simulink model "XM7p_new"  (R2024a)
settings: Solver=ode4  StartTime=0.0  StopTime=60  RelTol=1e-3
model workspace (MAT data in the model file):
  a_value = 1
undefined symbols (not defined in the file or in its folder): a, b, c_pol, dt, traj_par, X, Y, Z
libraries: sm_lib x280, nesl_utility x109, simulink x14
(part 1 of 6)
settings Model: Creator=asus  LastModifiedBy=17599
settings DebuggingCC: UnconnectedInputMsg=warning  UnconnectedOutputMsg=warning  UnconnectedLineMsg=warning
settings ModelReferenceCC: EnableRefExpFcnMdlSchedulingChecks=on
settings RTWCC: GPUComputeCapability=3.5  DLArmComputeVersion=19.05
settings ExplorerConfigSet: InternalSimMechanicsExplorerSettings="<ExplorerConfiguration><canonicalview>default</canonicalview><AnimationSetting><BasePlaybackSpeed>1.0</BasePlaybackSpeed><PlaybackSpeedFactor>1.0</PlaybackSpeedFactor></AnimationSetting><TilePanel><TileInfo><Tiles Columns=\"1\" Count=\"1\" Rows=\"1\"><Column Weight=\"1\"/><Row Weight=\"1\"/><Tile Height=\"1\" Width=\"1\" X=\"0\" Y=\"0\"/></Tiles></TileInfo><SceneInfo><SceneViewer><BGColor><R>0.60000002384185791</R><G>0.60000002384185791</G><B>0.60000002384185791</B></BGColor><Camera><DoPerspective>off</DoPerspective><Position><X>0.201838941505270653</X><Y>-1.16911856832824412</Y><Z>0.702483401800660268</Z></Position><Center><X>0.1539467503897545</X><Y>0.000995467000701073627</Y><Z>0.7153569470392378</Z></Center><Up><X>0.00490593321745084673</X><Y>-0.0108003862646076643</Y><Z>0.999929639262584158</Z></Up><ViewLimDist>1</ViewLimDist><YLim>0.987066108097597317</YLim><XLim>1.59392897455760174</XLim></Camera></SceneViewer></SceneInfo></TilePanel><MechEditorPanel><Cameras/><GfxPanelCameraMap/><VideoCreator><PlaybackSpeedRatio>1.0</PlaybackSpeedRatio><FrameRate>30</FrameRate><VideoFormat>MPEG-4</VideoFormat><FrameSize>auto</FrameSize></VideoCreator></MechEditorPanel></ExplorerConfiguration>"

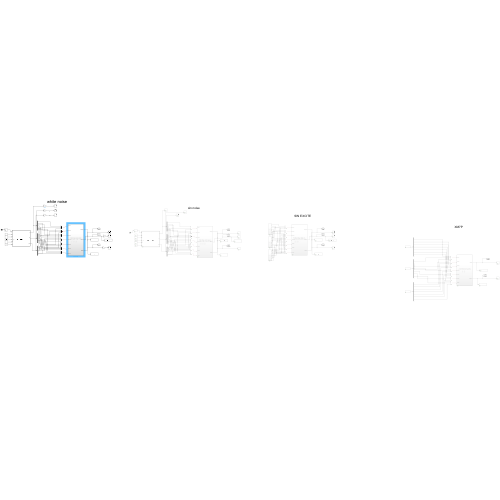
[thumbnail: Simulink's stored preview of the top-level diagram]
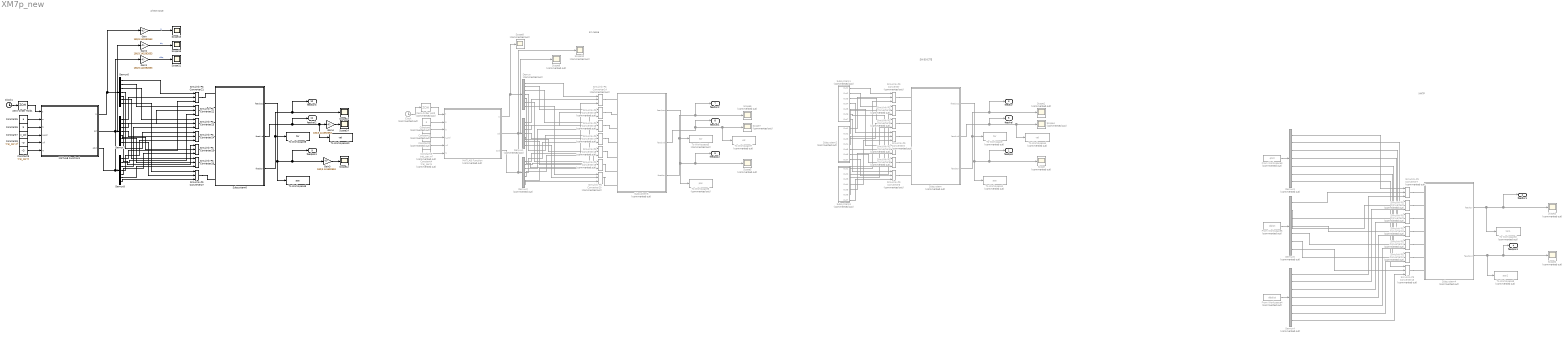
== system XM7p_new ==
  note: SIN EXCITE
  note: XM7P
  note: sin noise
  note: white noise
  Clock : Clock  Commented=on
  Clock1 : Clock
  Constant : Constant  Commented=on  Value=a  VectorParams1D=off
  Constant1 : Constant  Commented=on  Value=b  VectorParams1D=off
  Constant2 : Constant  Commented=on  Value=c_pol  VectorParams1D=off
  Constant3 : Constant  Commented=on  Value=traj_par.wf  VectorParams1D=off
  Constant4 : Constant  Commented=on  Value=traj_par.N  VectorParams1D=off
  Constant5 : Constant  Value=a  VectorParams1D=off
  Constant6 : Constant  Value=b  VectorParams1D=off
  Constant7 : Constant  Value=c_pol  VectorParams1D=off
  Constant8 : Constant  Value=traj_par.wf  VectorParams1D=off
  Constant9 : Constant  Value=traj_par.N  VectorParams1D=off
  Demux{,1..5} (6 alike) : Demux  Commented=on  Outputs=7
  Demux6 : Demux  Outputs=7
  Demux7 : Demux  Outputs=7
  Demux8 : Demux  Outputs=7
  From Workspace3 : FromWorkspace  Commented=on  VariableName=qlist  SampleTime=dt
  From Workspace4 : FromWorkspace  Commented=on  VariableName=ddqlist  SampleTime=dt
  From Workspace5 : FromWorkspace  Commented=on  VariableName=dqlist  SampleTime=dt
  Gain{,1..4} (5 alike) : Gain  Gain=180/3.141592653
  MATLAB Function : MATLAB Function  Commented=on  TreatAsAtomicUnit=on
  MATLAB Function1 : MATLAB Function  TreatAsAtomicUnit=on
  Scope{,1..10} (11 alike) : Scope  Commented=on
  Scope{11..16} (6 alike) : Scope
  Simulink-PS Converter{,1..20} (21 alike) : nesl_utility/Simulink-PS Converter  Commented=on  PhysicalDomain=network_engine_domain  SubClassName=ps_input  LeftPortType=input  RightPortType=output  PseudoPeriodic=off  Frequencies=[]  NoiseDistribution=none  NoiseParameters=[]  Unit=rad  AffineConversion=off  FilteringAndDerivatives=provide  SimscapeFilterOrder=2  InputFilterTimeConstant=0.001  UdotUserProvided=2
  Simulink-PS Converter{21..27} (7 alike) : nesl_utility/Simulink-PS Converter  PhysicalDomain=network_engine_domain  SubClassName=ps_input  LeftPortType=input  RightPortType=output  PseudoPeriodic=off  Frequencies=[]  NoiseDistribution=none  NoiseParameters=[]  Unit=rad  AffineConversion=off  FilteringAndDerivatives=provide  SimscapeFilterOrder=2  InputFilterTimeConstant=0.001  UdotUserProvided=2
  Subsystem : Subsystem  Commented=on
  Subsystem1 : Subsystem  Commented=on
  Subsystem2 : Subsystem  Commented=on
  Subsystem3 : Subsystem  Commented=on
  Subsystem4 : Subsystem  Commented=on
  Subsystem5 : Subsystem  Commented=on
  Subsystem6 : Subsystem
  To Workspace : ToWorkspace  Commented=on  VariableName=tor  SampleTime=-1
      settings: Save2DSignal=2-D array (concatenate along first dimension)
  To Workspace1 : ToWorkspace  Commented=on  VariableName=pos  SampleTime=-1
      settings: Save2DSignal=2-D array (concatenate along first dimension)
  To Workspace10 : ToWorkspace  VariableName=vel  SampleTime=-1
      settings: Save2DSignal=2-D array (concatenate along first dimension)
  To Workspace2 : ToWorkspace  Commented=on  VariableName=tor1  SampleTime=-1
      settings: Save2DSignal=2-D array (concatenate along first dimension)
  To Workspace3 : ToWorkspace  Commented=on  VariableName=pos1  SampleTime=-1
      settings: Save2DSignal=2-D array (concatenate along first dimension)
  To Workspace4 : ToWorkspace  Commented=on  VariableName=vel  SampleTime=-1
      settings: Save2DSignal=2-D array (concatenate along first dimension)
  To Workspace5 : ToWorkspace  Commented=on  VariableName=tor  SampleTime=-1
      settings: Save2DSignal=2-D array (concatenate along first dimension)
  To Workspace6 : ToWorkspace  Commented=on  VariableName=pos  SampleTime=-1
      settings: Save2DSignal=2-D array (concatenate along first dimension)
  To Workspace7 : ToWorkspace  Commented=on  VariableName=vel  SampleTime=-1
      settings: Save2DSignal=2-D array (concatenate along first dimension)
  To Workspace8 : ToWorkspace  VariableName=tor  SampleTime=-1
      settings: Save2DSignal=2-D array (concatenate along first dimension)
  To Workspace9 : ToWorkspace  VariableName=pos  SampleTime=-1
      settings: Save2DSignal=2-D array (concatenate along first dimension)
  Zero-Order Hold : ZeroOrderHold  Commented=on  SampleTime=0.001
  Zero-Order Hold1 : ZeroOrderHold  SampleTime=0.001
  feedpos : Outport  Unit=rad
  feedtor1 : Outport  Port=2  Unit=N*m
  feedtor : Outport  Port=3  Unit=N*m
  feedpos1 : Outport  Port=4  Unit=rad
  feedvel : Outport  Port=5  Unit=rad/s
  feedpos2 : Outport  Port=6  Unit=rad
  feedtor2 : Outport  Port=7  Unit=N*m
  feedvel1 : Outport  Port=8  Unit=rad/s
  feedpos3 : Outport  Port=9  Unit=rad
  feedtor3 : Outport  Port=10  Unit=N*m
  feedvel2 : Outport  Port=11  Unit=rad/s
  wires:
  Subsystem/3(feedtor) -> feedtor/1, Scope1/1, To Workspace/1
  Subsystem/1(feedpos) -> To Workspace1/1, feedpos/1, Scope/1
  Subsystem1/1(Out1) -> Simulink-PS Converter/1
  Subsystem1/2(Out2) -> Simulink-PS Converter1/1
  Subsystem1/3(Out3) -> Simulink-PS Converter2/1
  Subsystem1/4(Out4) -> Simulink-PS Converter3/1
  Subsystem1/5(Out5) -> Simulink-PS Converter4/1
  Subsystem1/6(Out6) -> Simulink-PS Converter5/1
  Subsystem1/7(Out7) -> Simulink-PS Converter6/1
  Subsystem2/1(Out1) -> Simulink-PS Converter/2
  Subsystem2/2(Out2) -> Simulink-PS Converter1/2
  Subsystem2/3(Out3) -> Simulink-PS Converter2/2
  Subsystem2/4(Out4) -> Simulink-PS Converter3/2
  Subsystem2/5(Out5) -> Simulink-PS Converter4/2
  Subsystem2/6(Out6) -> Simulink-PS Converter5/2
  Subsystem2/7(Out7) -> Simulink-PS Converter6/2
  Subsystem3/1(Out1) -> Simulink-PS Converter/3
  Subsystem3/2(Out2) -> Simulink-PS Converter1/3
  Subsystem3/3(Out3) -> Simulink-PS Converter2/3
  Subsystem3/4(Out4) -> Simulink-PS Converter3/3
  Subsystem3/5(Out5) -> Simulink-PS Converter4/3
  Subsystem3/6(Out6) -> Simulink-PS Converter5/3
  Subsystem3/7(Out7) -> Simulink-PS Converter6/3
  Demux3/5 -> Simulink-PS Converter11/1
  Demux4/6 -> Simulink-PS Converter12/3
  Demux5/2 -> Simulink-PS Converter8/2
  Demux4/5 -> Simulink-PS Converter11/3
  Demux5/7 -> Simulink-PS Converter13/2
  Demux5/3 -> Simulink-PS Converter9/2
  Demux4/7 -> Simulink-PS Converter13/3
  Demux3/2 -> Simulink-PS Converter8/1
  Demux3/4 -> Simulink-PS Converter10/1
  From Workspace5/1 -> Demux5/1
  Demux4/3 -> Simulink-PS Converter9/3
  Demux5/5 -> Simulink-PS Converter11/2
  Demux3/3 -> Simulink-PS Converter9/1
  Subsystem4/2(feedpos) -> Scope2/1, feedpos1/1, To Workspace3/1
  Demux4/2 -> Simulink-PS Converter8/3
  Demux4/1 -> Simulink-PS Converter7/3
  Demux4/4 -> Simulink-PS Converter10/3
  Demux3/6 -> Simulink-PS Converter12/1
  From Workspace3/1 -> Demux3/1
  Demux5/6 -> Simulink-PS Converter12/2
  From Workspace4/1 -> Demux4/1
  Demux5/4 -> Simulink-PS Converter10/2
  Demux3/1 -> Simulink-PS Converter7/1
  Demux5/1 -> Simulink-PS Converter7/2
  Subsystem4/1(feedtor) -> To Workspace2/1, feedtor1/1, Scope3/1
  Demux3/7 -> Simulink-PS Converter13/1
  Subsystem/2(feedvel) -> feedvel/1, To Workspace4/1, Scope4/1
  Subsystem5/2(feedvel) -> feedvel1/1, To Workspace7/1, Scope7/1
  Subsystem5/1(feedpos) -> To Workspace6/1, feedpos2/1, Scope5/1
  Subsystem5/3(feedtor) -> feedtor2/1, Scope6/1, To Workspace5/1
  Clock/1 -> Zero-Order Hold/1
  Constant/1 -> MATLAB Function/2(a)
  Constant1/1 -> MATLAB Function/3(b)
  Constant2/1 -> MATLAB Function/4(c_pol)
  Constant3/1 -> MATLAB Function/5(wf)
  Constant4/1 -> MATLAB Function/6(N)
  Demux/1 -> Simulink-PS Converter14/1
  Demux/2 -> Simulink-PS Converter15/1
  Demux/3 -> Simulink-PS Converter16/1
  Demux/4 -> Simulink-PS Converter17/1
  Demux/5 -> Simulink-PS Converter18/1
  Demux/6 -> Simulink-PS Converter19/1
  Demux/7 -> Simulink-PS Converter20/1
  Demux1/1 -> Simulink-PS Converter14/2
  Demux1/2 -> Simulink-PS Converter15/2
  Demux1/3 -> Simulink-PS Converter16/2
  Demux1/4 -> Simulink-PS Converter17/2
  Demux1/5 -> Simulink-PS Converter18/2
  Demux1/6 -> Simulink-PS Converter19/2
  Demux1/7 -> Simulink-PS Converter20/2
  Demux2/1 -> Simulink-PS Converter14/3
  Demux2/2 -> Simulink-PS Converter15/3
  Demux2/3 -> Simulink-PS Converter16/3
  Demux2/4 -> Simulink-PS Converter17/3
  Demux2/5 -> Simulink-PS Converter18/3
  Demux2/6 -> Simulink-PS Converter19/3
  Demux2/7 -> Simulink-PS Converter20/3
  MATLAB Function/1(q) -> Scope8/1, Demux/1
  MATLAB Function/2(qd) -> Scope9/1, Demux1/1
  MATLAB Function/3(q2d) -> Scope10/1, Demux2/1
  Zero-Order Hold/1 -> MATLAB Function/1(t)
  Demux7/3 -> Simulink-PS Converter23/2
  Demux7/4 -> Simulink-PS Converter24/2
  Constant8/1 -> MATLAB Function1/5(wf)
  Subsystem6/3(feedtor) -> feedtor3/1, Scope13/1, To Workspace8/1
  Clock1/1 -> Zero-Order Hold1/1
  Constant9/1 -> MATLAB Function1/6(N)
  Demux6/7 -> Simulink-PS Converter27/1
  Demux6/6 -> Simulink-PS Converter26/1
  Demux6/4 -> Simulink-PS Converter24/1
  Demux7/1 -> Simulink-PS Converter21/2
  Demux6/5 -> Simulink-PS Converter25/1
  Demux7/5 -> Simulink-PS Converter25/2
  Subsystem6/1(feedpos) -> To Workspace9/1, feedpos3/1, Gain3/1
  Zero-Order Hold1/1 -> MATLAB Function1/1(t)
  MATLAB Function1/2(qd) -> Gain2/1, Demux7/1
  Demux8/1 -> Simulink-PS Converter21/3
  Demux6/2 -> Simulink-PS Converter22/1
  MATLAB Function1/3(q2d) -> Gain1/1, Demux8/1
  Subsystem6/2(feedvel) -> feedvel2/1, To Workspace10/1, Gain4/1
  Demux8/7 -> Simulink-PS Converter27/3
  Demux6/1 -> Simulink-PS Converter21/1
  Constant7/1 -> MATLAB Function1/4(c_pol)
  MATLAB Function1/1(q) -> Gain/1, Demux6/1
  Demux8/2 -> Simulink-PS Converter22/3
  Demux8/3 -> Simulink-PS Converter23/3
  Demux8/5 -> Simulink-PS Converter25/3
  Demux8/6 -> Simulink-PS Converter26/3
  Demux7/2 -> Simulink-PS Converter22/2
  Constant5/1 -> MATLAB Function1/2(a)
  Demux7/7 -> Simulink-PS Converter27/2
  Constant6/1 -> MATLAB Function1/3(b)
  Demux6/3 -> Simulink-PS Converter23/1
  Demux8/4 -> Simulink-PS Converter24/3
  Demux7/6 -> Simulink-PS Converter26/2
  Gain/1 -> Scope15/1  "q"
  Gain1/1 -> Scope11/1  "ddq"
  Gain2/1 -> Scope16/1  "dq"
  Gain3/1 -> Scope12/1
  Gain4/1 -> Scope14/1
  connections:
  Simulink-PS Converter/RConn1 -- Subsystem/LConn1
  Simulink-PS Converter6/RConn1 -- Subsystem/LConn7
  Simulink-PS Converter4/RConn1 -- Subsystem/LConn5
  Simulink-PS Converter2/RConn1 -- Subsystem/LConn3
  Simulink-PS Converter1/RConn1 -- Subsystem/LConn2
  Simulink-PS Converter5/RConn1 -- Subsystem/LConn6
  Simulink-PS Converter3/RConn1 -- Subsystem/LConn4
  Simulink-PS Converter10/RConn1 -- Subsystem4/LConn4
  Simulink-PS Converter13/RConn1 -- Subsystem4/LConn7
  Simulink-PS Converter9/RConn1 -- Subsystem4/LConn3
  Simulink-PS Converter8/RConn1 -- Subsystem4/LConn2
  Simulink-PS Converter12/RConn1 -- Subsystem4/LConn6
  Simulink-PS Converter7/RConn1 -- Subsystem4/LConn1
  Simulink-PS Converter11/RConn1 -- Subsystem4/LConn5
  Simulink-PS Converter14/RConn1 -- Subsystem5/LConn1
  Simulink-PS Converter20/RConn1 -- Subsystem5/LConn7
  Simulink-PS Converter17/RConn1 -- Subsystem5/LConn4
  Simulink-PS Converter18/RConn1 -- Subsystem5/LConn5
  Simulink-PS Converter19/RConn1 -- Subsystem5/LConn6
  Simulink-PS Converter15/RConn1 -- Subsystem5/LConn2
  Simulink-PS Converter16/RConn1 -- Subsystem5/LConn3
  Simulink-PS Converter26/RConn1 -- Subsystem6/LConn6
  Simulink-PS Converter22/RConn1 -- Subsystem6/LConn2
  Simulink-PS Converter27/RConn1 -- Subsystem6/LConn7
  Simulink-PS Converter24/RConn1 -- Subsystem6/LConn4
  Simulink-PS Converter23/RConn1 -- Subsystem6/LConn3
  Simulink-PS Converter25/RConn1 -- Subsystem6/LConn5
  Simulink-PS Converter21/RConn1 -- Subsystem6/LConn1

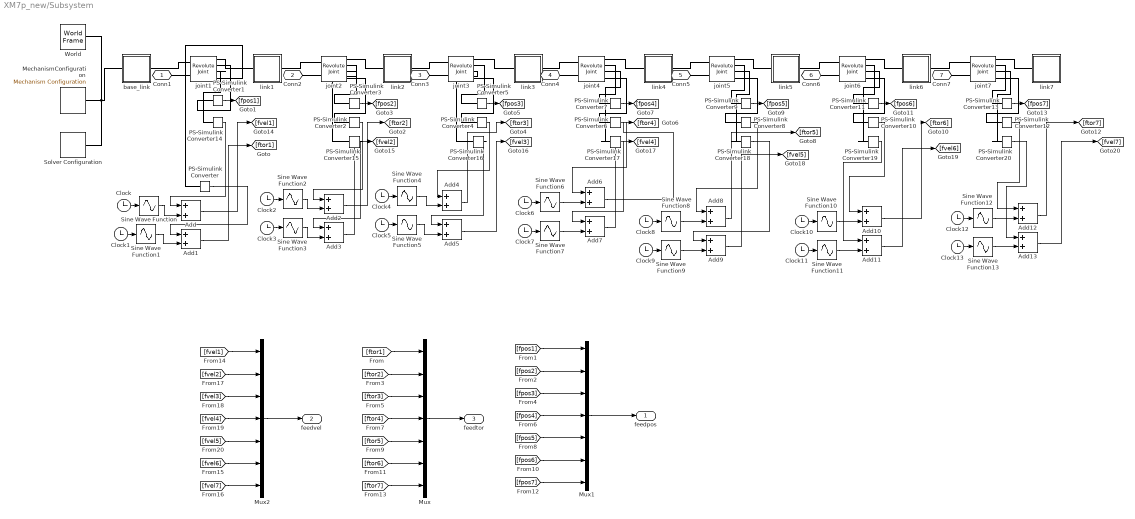
== system XM7p_new/Subsystem ==
  Add{,1..13} (14 alike) : Sum
  Clock{,1..13} (14 alike) : Clock
  MechanismConfiguration : sm_lib/Utilities/Mechanism Configuration  UniformGravity=Constant  GravityVector=[0 0 -9.80665]  GravityVectorUnits=m/s^2  LinearizationDelta=0.001  JointModeTransitionNonlinearIterations=2
  Mux : Mux  Inputs=7
  Mux1 : Mux  Inputs=7
  Mux2 : Mux  Inputs=7
  PS-Simulink Converter{,2,4,6,8,10,12} (7 alike) : nesl_utility/PS-Simulink Converter  PhysicalDomain=network_engine_domain  SubClassName=ps_output  LeftPortType=input  RightPortType=output  PseudoPeriodic=off  Frequencies=[]  VectorFormat=1-D array  Unit=N*m  AffineConversion=off
  PS-Simulink Converter{1,3,5,7,9,11,13} (7 alike) : nesl_utility/PS-Simulink Converter  PhysicalDomain=network_engine_domain  SubClassName=ps_output  LeftPortType=input  RightPortType=output  PseudoPeriodic=off  Frequencies=[]  VectorFormat=1-D array  Unit=rad  AffineConversion=off
  PS-Simulink Converter{14..20} (7 alike) : nesl_utility/PS-Simulink Converter  PhysicalDomain=network_engine_domain  SubClassName=ps_output  LeftPortType=input  RightPortType=output  PseudoPeriodic=off  Frequencies=[]  VectorFormat=1-D array  Unit=rad/s  AffineConversion=off
  Sine Wave Function{,1,3..5} (5 alike) : Sin  TimeSource=Use external signal  Amplitude=0.05  Frequency=10  SampleTime=0
  Sine Wave Function{6..11} (6 alike) : Sin  TimeSource=Use external signal  Amplitude=0.03  Frequency=10  SampleTime=0
  Sine Wave Function12 : Sin  TimeSource=Use external signal  Amplitude=0.02  Frequency=10  SampleTime=0
  Sine Wave Function13 : Sin  TimeSource=Use external signal  Amplitude=0.02  Frequency=10  SampleTime=0
  Sine Wave Function2 : Sin  TimeSource=Use external signal  Amplitude=0.05  SampleTime=0
  Solver Configuration : nesl_utility/Solver Configuration  PhysicalDomain=network_engine_domain  SubClassName=solver  LeftPortType=input  RightPortType=generic  Tones=[]  Harmonics=[]  SimulateNoise=off  Profile=off  UseLocalSampling=off  EnableSwitchedLinearOptims=on  FrequencyDomain=off  UseCCode=off  RelTol=0.001  AbsTol=1e-06  MinStep=1e-09  ToWorkspace=off  RevertToSquareIcSolve=off  NumHomotopyIterations=100  PhasorMode=off  PhasorModeNumHarmonics=1  ConsistencySolver=NEWTON_FTOL  IndexReductionMethod=DerivativeReplacement  DoDC=off  ResidualTolerance=1e-09  ConsistencyTolSource=GLOBAL  ConsistencyAbsTol=0.001  ConsistencyRelTol=0.001  ConsistencyTolFactor=0.001  UseLocalSolver=off  LocalSolverChoice=NE_BACKWARD_EULER_ADVANCER  ResolveIndetEquations=on  FunctionEvalNumThread=1  LocalSolverSampleTime=0.001  DoFixedCost=off  MaxNonlinIter=3  MaxModeIter=2  ComputeImpulses=off  ImpulseIterations=2  LinearAlgebra=auto  LinearAlgebraNumThread=0  EquationFormulation=NE_TIME_EF  DelaysMemoryBudget=1024  AutomaticFiltering=on  FilteringTimeConstant=0.001  PartitionStorageMethod=AS_NEEDED  PartitionMemoryBudget=1024  PartitionMethod=ROBUST  MultibodyUseLocalSolver=off  MultibodyLocalSolverChoice=ODE1  MultibodyLocalSolverSampleTime=0.001
  World : sm_lib/Frames and Transforms/World Frame
  base_link : Subsystem
  joint1 : sm_lib/Joints/Revolute Joint  JointMode=Normal  CompositeWrenchDir=FollowerOnBase  CompositeWrenchFrame=BaseFrame  SenseConstraintForce=off  SenseConstraintTorque=off  SenseTotalForce=off  SenseTotalTorque=off  PositionTargetSpecify=off  PositionTargetPriority=High  PositionTargetValue=0  PositionTargetValueUnits=deg  VelocityTargetSpecify=off  VelocityTargetPriority=High  VelocityTargetValue=0  VelocityTargetValueUnits=deg/s  EquilibriumPosition=0  EquilibriumPositionUnits=deg  SpringStiffness=0  SpringStiffnessUnits=N*m/deg  DampingCoefficient=0  DampingCoefficientUnits=kg*m^2/(rad*s)  LowerLimitSpecify=on  LowerLimitBound=-3.1067  LowerLimitBoundUnits=rad  LowerLimitStiffness=1e4  LowerLimitStiffnessUnits=N*m/deg  LowerLimitDamping=10  LowerLimitDampingUnits=N*m/(deg/s)  LowerLimitTransitionRegionWidth=0.1  LowerLimitTransitionRegionWidthUnits=deg  UpperLimitSpecify=on  UpperLimitBound=3.1067  UpperLimitBoundUnits=rad  UpperLimitStiffness=1e4  UpperLimitStiffnessUnits=N*m/deg  UpperLimitDamping=10  UpperLimitDampingUnits=N*m/(deg/s)  UpperLimitTransitionRegionWidth=0.1  UpperLimitTransitionRegionWidthUnits=deg  TorqueActuationMode=ComputedTorque  MotionActuationMode=InputMotion  SensePosition=on  SenseVelocity=on  SenseAcceleration=off  SenseTorqueForce=on  SenseLowerLimitTorqueForce=off  SenseUpperLimitTorqueForce=off
  joint2 : sm_lib/Joints/Revolute Joint  JointMode=Normal  CompositeWrenchDir=FollowerOnBase  CompositeWrenchFrame=BaseFrame  SenseConstraintForce=off  SenseConstraintTorque=off  SenseTotalForce=off  SenseTotalTorque=off  PositionTargetSpecify=off  PositionTargetPriority=High  PositionTargetValue=0  PositionTargetValueUnits=deg  VelocityTargetSpecify=off  VelocityTargetPriority=High  VelocityTargetValue=0  VelocityTargetValueUnits=deg/s  EquilibriumPosition=0  EquilibriumPositionUnits=deg  SpringStiffness=0  SpringStiffnessUnits=N*m/deg  DampingCoefficient=0  DampingCoefficientUnits=kg*m^2/(rad*s)  LowerLimitSpecify=on  LowerLimitBound=-2.09  LowerLimitBoundUnits=rad  LowerLimitStiffness=1e4  LowerLimitStiffnessUnits=N*m/deg  LowerLimitDamping=10  LowerLimitDampingUnits=N*m/(deg/s)  LowerLimitTransitionRegionWidth=0.1  LowerLimitTransitionRegionWidthUnits=deg  UpperLimitSpecify=on  UpperLimitBound=2.09  UpperLimitBoundUnits=rad  UpperLimitStiffness=1e4  UpperLimitStiffnessUnits=N*m/deg  UpperLimitDamping=10  UpperLimitDampingUnits=N*m/(deg/s)  UpperLimitTransitionRegionWidth=0.1  UpperLimitTransitionRegionWidthUnits=deg  TorqueActuationMode=ComputedTorque  MotionActuationMode=InputMotion  SensePosition=on  SenseVelocity=on  SenseAcceleration=off  SenseTorqueForce=on  SenseLowerLimitTorqueForce=off  SenseUpperLimitTorqueForce=off
  joint3 : sm_lib/Joints/Revolute Joint  JointMode=Normal  CompositeWrenchDir=FollowerOnBase  CompositeWrenchFrame=BaseFrame  SenseConstraintForce=off  SenseConstraintTorque=off  SenseTotalForce=off  SenseTotalTorque=off  PositionTargetSpecify=off  PositionTargetPriority=High  PositionTargetValue=0  PositionTargetValueUnits=deg  VelocityTargetSpecify=off  VelocityTargetPriority=High  VelocityTargetValue=0  VelocityTargetValueUnits=deg/s  EquilibriumPosition=0  EquilibriumPositionUnits=deg  SpringStiffness=0  SpringStiffnessUnits=N*m/deg  DampingCoefficient=0  DampingCoefficientUnits=kg*m^2/(rad*s)  LowerLimitSpecify=on  LowerLimitBound=-3.1067  LowerLimitBoundUnits=rad  LowerLimitStiffness=1e4  LowerLimitStiffnessUnits=N*m/deg  LowerLimitDamping=10  LowerLimitDampingUnits=N*m/(deg/s)  LowerLimitTransitionRegionWidth=0.1  LowerLimitTransitionRegionWidthUnits=deg  UpperLimitSpecify=on  UpperLimitBound=3.1067  UpperLimitBoundUnits=rad  UpperLimitStiffness=1e4  UpperLimitStiffnessUnits=N*m/deg  UpperLimitDamping=10  UpperLimitDampingUnits=N*m/(deg/s)  UpperLimitTransitionRegionWidth=0.1  UpperLimitTransitionRegionWidthUnits=deg  TorqueActuationMode=ComputedTorque  MotionActuationMode=InputMotion  SensePosition=on  SenseVelocity=on  SenseAcceleration=off  SenseTorqueForce=on  SenseLowerLimitTorqueForce=off  SenseUpperLimitTorqueForce=off
  joint4 : sm_lib/Joints/Revolute Joint  JointMode=Normal  CompositeWrenchDir=FollowerOnBase  CompositeWrenchFrame=BaseFrame  SenseConstraintForce=off  SenseConstraintTorque=off  SenseTotalForce=off  SenseTotalTorque=off  PositionTargetSpecify=off  PositionTargetPriority=High  PositionTargetValue=0  PositionTargetValueUnits=deg  VelocityTargetSpecify=off  VelocityTargetPriority=High  VelocityTargetValue=0  VelocityTargetValueUnits=deg/s  EquilibriumPosition=0  EquilibriumPositionUnits=deg  SpringStiffness=0  SpringStiffnessUnits=N*m/deg  DampingCoefficient=0  DampingCoefficientUnits=kg*m^2/(rad*s)  LowerLimitSpecify=on  LowerLimitBound=-2.5307  LowerLimitBoundUnits=rad  LowerLimitStiffness=1e4  LowerLimitStiffnessUnits=N*m/deg  LowerLimitDamping=10  LowerLimitDampingUnits=N*m/(deg/s)  LowerLimitTransitionRegionWidth=0.1  LowerLimitTransitionRegionWidthUnits=deg  UpperLimitSpecify=on  UpperLimitBound=1.0472  UpperLimitBoundUnits=rad  UpperLimitStiffness=1e4  UpperLimitStiffnessUnits=N*m/deg  UpperLimitDamping=10  UpperLimitDampingUnits=N*m/(deg/s)  UpperLimitTransitionRegionWidth=0.1  UpperLimitTransitionRegionWidthUnits=deg  TorqueActuationMode=ComputedTorque  MotionActuationMode=InputMotion  SensePosition=on  SenseVelocity=on  SenseAcceleration=off  SenseTorqueForce=on  SenseLowerLimitTorqueForce=off  SenseUpperLimitTorqueForce=off
  joint5 : sm_lib/Joints/Revolute Joint  JointMode=Normal  CompositeWrenchDir=FollowerOnBase  CompositeWrenchFrame=BaseFrame  SenseConstraintForce=off  SenseConstraintTorque=off  SenseTotalForce=off  SenseTotalTorque=off  PositionTargetSpecify=off  PositionTargetPriority=High  PositionTargetValue=0  PositionTargetValueUnits=deg  VelocityTargetSpecify=off  VelocityTargetPriority=High  VelocityTargetValue=0  VelocityTargetValueUnits=deg/s  EquilibriumPosition=0  EquilibriumPositionUnits=deg  SpringStiffness=0  SpringStiffnessUnits=N*m/deg  DampingCoefficient=0  DampingCoefficientUnits=kg*m^2/(rad*s)  LowerLimitSpecify=on  LowerLimitBound=-3.1067  LowerLimitBoundUnits=rad  LowerLimitStiffness=1e4  LowerLimitStiffnessUnits=N*m/deg  LowerLimitDamping=10  LowerLimitDampingUnits=N*m/(deg/s)  LowerLimitTransitionRegionWidth=0.1  LowerLimitTransitionRegionWidthUnits=deg  UpperLimitSpecify=on  UpperLimitBound=3.1067  UpperLimitBoundUnits=rad  UpperLimitStiffness=1e4  UpperLimitStiffnessUnits=N*m/deg  UpperLimitDamping=10  UpperLimitDampingUnits=N*m/(deg/s)  UpperLimitTransitionRegionWidth=0.1  UpperLimitTransitionRegionWidthUnits=deg  TorqueActuationMode=ComputedTorque  MotionActuationMode=InputMotion  SensePosition=on  SenseVelocity=on  SenseAcceleration=off  SenseTorqueForce=on  SenseLowerLimitTorqueForce=off  SenseUpperLimitTorqueForce=off
  joint6 : sm_lib/Joints/Revolute Joint  JointMode=Normal  CompositeWrenchDir=FollowerOnBase  CompositeWrenchFrame=BaseFrame  SenseConstraintForce=off  SenseConstraintTorque=off  SenseTotalForce=off  SenseTotalTorque=off  PositionTargetSpecify=off  PositionTargetPriority=High  PositionTargetValue=0  PositionTargetValueUnits=deg  VelocityTargetSpecify=off  VelocityTargetPriority=High  VelocityTargetValue=0  VelocityTargetValueUnits=deg/s  EquilibriumPosition=0  EquilibriumPositionUnits=deg  SpringStiffness=0  SpringStiffnessUnits=N*m/deg  DampingCoefficient=0  DampingCoefficientUnits=kg*m^2/(rad*s)  LowerLimitSpecify=on  LowerLimitBound=-1.0472  LowerLimitBoundUnits=rad  LowerLimitStiffness=1e4  LowerLimitStiffnessUnits=N*m/deg  LowerLimitDamping=10  LowerLimitDampingUnits=N*m/(deg/s)  LowerLimitTransitionRegionWidth=0.1  LowerLimitTransitionRegionWidthUnits=deg  UpperLimitSpecify=on  UpperLimitBound=1.0472  UpperLimitBoundUnits=rad  UpperLimitStiffness=1e4  UpperLimitStiffnessUnits=N*m/deg  UpperLimitDamping=10  UpperLimitDampingUnits=N*m/(deg/s)  UpperLimitTransitionRegionWidth=0.1  UpperLimitTransitionRegionWidthUnits=deg  TorqueActuationMode=ComputedTorque  MotionActuationMode=InputMotion  SensePosition=on  SenseVelocity=on  SenseAcceleration=off  SenseTorqueForce=on  SenseLowerLimitTorqueForce=off  SenseUpperLimitTorqueForce=off
  joint7 : sm_lib/Joints/Revolute Joint  JointMode=Normal  CompositeWrenchDir=FollowerOnBase  CompositeWrenchFrame=BaseFrame  SenseConstraintForce=off  SenseConstraintTorque=off  SenseTotalForce=off  SenseTotalTorque=off  PositionTargetSpecify=off  PositionTargetPriority=High  PositionTargetValue=0  PositionTargetValueUnits=deg  VelocityTargetSpecify=off  VelocityTargetPriority=High  VelocityTargetValue=0  VelocityTargetValueUnits=deg/s  EquilibriumPosition=0  EquilibriumPositionUnits=deg  SpringStiffness=0  SpringStiffnessUnits=N*m/deg  DampingCoefficient=0  DampingCoefficientUnits=kg*m^2/(rad*s)  LowerLimitSpecify=on  LowerLimitBound=-1.5708  LowerLimitBoundUnits=rad  LowerLimitStiffness=1e4  LowerLimitStiffnessUnits=N*m/deg  LowerLimitDamping=10  LowerLimitDampingUnits=N*m/(deg/s)  LowerLimitTransitionRegionWidth=0.1  LowerLimitTransitionRegionWidthUnits=deg  UpperLimitSpecify=on  UpperLimitBound=1.5708  UpperLimitBoundUnits=rad  UpperLimitStiffness=1e4  UpperLimitStiffnessUnits=N*m/deg  UpperLimitDamping=10  UpperLimitDampingUnits=N*m/(deg/s)  UpperLimitTransitionRegionWidth=0.1  UpperLimitTransitionRegionWidthUnits=deg  TorqueActuationMode=ComputedTorque  MotionActuationMode=InputMotion  SensePosition=on  SenseVelocity=on  SenseAcceleration=off  SenseTorqueForce=on  SenseLowerLimitTorqueForce=off  SenseUpperLimitTorqueForce=off
  link1 : Subsystem
  link2 : Subsystem
  link3 : Subsystem
  link4 : Subsystem
  link5 : Subsystem
  link6 : Subsystem
  link7 : Subsystem
  Conn1 : PMIOPort  Side=Left
  Conn2 : PMIOPort  Port=2  Side=Left
  Conn3 : PMIOPort  Port=3  Side=Left
  Conn4 : PMIOPort  Port=4  Side=Left
  Conn5 : PMIOPort  Port=5  Side=Left
  Conn6 : PMIOPort  Port=6  Side=Left
  Conn7 : PMIOPort  Port=7  Side=Left
  feedpos : Outport  Unit=rad
  feedvel : Outport  Port=2  Unit=rad/s
  feedtor : Outport  Port=3  Unit=N*m
  wires:
  [fpos5] -> Mux1/5
  PS-Simulink Converter1/1 -> [fpos1]
  [fpos1] -> Mux1/1
  PS-Simulink Converter11/1 -> [fpos6]
  PS-Simulink Converter10/1 -> Add10/1
  Mux1/1 -> feedpos/1
  [ftor3] -> Mux/3
  PS-Simulink Converter13/1 -> [fpos7]
  PS-Simulink Converter4/1 -> Add4/1
  Mux/1 -> feedtor/1
  PS-Simulink Converter/1 -> Add1/1
  PS-Simulink Converter3/1 -> [fpos2]
  PS-Simulink Converter9/1 -> [fpos5]
  PS-Simulink Converter6/1 -> Add6/1
  PS-Simulink Converter7/1 -> [fpos4]
  PS-Simulink Converter12/1 -> Add12/1
  [fpos2] -> Mux1/2
  PS-Simulink Converter8/1 -> Add8/1
  [ftor4] -> Mux/4
  [fpos6] -> Mux1/6
  [ftor2] -> Mux/2
  [fpos7] -> Mux1/7
  [ftor1] -> Mux/1
  [ftor6] -> Mux/6
  [fpos4] -> Mux1/4
  [fpos3] -> Mux1/3
  [ftor7] -> Mux/7
  [ftor5] -> Mux/5
  [fvel5] -> Mux2/5
  [fvel1] -> Mux2/1
  [fvel7] -> Mux2/7
  [fvel3] -> Mux2/3
  [fvel6] -> Mux2/6
  [fvel4] -> Mux2/4
  [fvel2] -> Mux2/2
  Mux2/1 -> feedvel/1
  PS-Simulink Converter17/1 -> Add7/1
  PS-Simulink Converter18/1 -> Add9/1
  PS-Simulink Converter19/1 -> Add11/1
  PS-Simulink Converter20/1 -> Add13/1
  Sine Wave Function/1 -> Add/2
  PS-Simulink Converter14/1 -> Add/1
  Add/1 -> [fvel1]
  Sine Wave Function1/1 -> Add1/2
  Add1/1 -> [ftor1]
  PS-Simulink Converter2/1 -> Add2/1
  Add3/1 -> [fvel2]
  Sine Wave Function2/1 -> Add2/2
  PS-Simulink Converter15/1 -> Add3/1
  Add2/1 -> [ftor2]
  Sine Wave Function3/1 -> Add3/2
  Clock/1 -> Sine Wave Function/1
  Clock1/1 -> Sine Wave Function1/1
  Clock2/1 -> Sine Wave Function2/1
  Clock3/1 -> Sine Wave Function3/1
  Clock5/1 -> Sine Wave Function5/1
  Sine Wave Function5/1 -> Add5/2
  Add5/1 -> [fvel3]
  PS-Simulink Converter16/1 -> Add5/1
  Clock4/1 -> Sine Wave Function4/1
  Sine Wave Function4/1 -> Add4/2
  Add4/1 -> [ftor3]
  PS-Simulink Converter5/1 -> [fpos3]
  Clock7/1 -> Sine Wave Function7/1
  Sine Wave Function7/1 -> Add7/2
  Clock6/1 -> Sine Wave Function6/1
  Sine Wave Function6/1 -> Add6/2
  Add6/1 -> [ftor4]
  Add7/1 -> [fvel4]
  Clock9/1 -> Sine Wave Function9/1
  Sine Wave Function9/1 -> Add9/2
  Clock8/1 -> Sine Wave Function8/1
  Sine Wave Function8/1 -> Add8/2
  Clock10/1 -> Sine Wave Function10/1
  Sine Wave Function10/1 -> Add10/2
  Sine Wave Function11/1 -> Add11/2
  Clock11/1 -> Sine Wave Function11/1
  Clock13/1 -> Sine Wave Function13/1
  Sine Wave Function13/1 -> Add13/2
  Sine Wave Function12/1 -> Add12/2
  Clock12/1 -> Sine Wave Function12/1
  Add8/1 -> [ftor5]
  Add9/1 -> [fvel5]
  Add10/1 -> [ftor6]
  Add11/1 -> [fvel6]
  Add12/1 -> [ftor7]
  Add13/1 -> [fvel7]
  connections:
  joint4/RConn1 -- link4/LConn1
  joint3/RConn2 -- PS-Simulink Converter5/LConn1
  joint5/RConn1 -- link5/LConn1
  joint1/RConn2 -- PS-Simulink Converter1/LConn1
  joint5/LConn1 -- link4/RConn1
  joint5/RConn2 -- PS-Simulink Converter9/LConn1
  joint2/RConn2 -- PS-Simulink Converter3/LConn1
  joint6/LConn2 -- Conn6/RConn1
  joint1/RConn1 -- link1/LConn1
  joint1/RConn4 -- PS-Simulink Converter/LConn1
  joint2/RConn4 -- PS-Simulink Converter2/LConn1
  joint7/RConn1 -- link7/LConn1
  joint4/RConn4 -- PS-Simulink Converter6/LConn1
  joint5/LConn2 -- Conn5/RConn1
  World/RConn1 -- MechanismConfiguration/RConn1 -- Solver Configuration/RConn1 -- base_link/LConn1
  joint2/LConn1 -- link1/RConn1
  joint7/RConn2 -- PS-Simulink Converter13/LConn1
  joint4/RConn2 -- PS-Simulink Converter7/LConn1
  joint2/RConn1 -- link2/LConn1
  joint7/LConn2 -- Conn7/RConn1
  joint6/RConn1 -- link6/LConn1
  joint6/LConn1 -- link5/RConn1
  joint7/LConn1 -- link6/RConn1
  base_link/RConn1 -- joint1/LConn1
  joint3/LConn2 -- Conn3/RConn1
  joint4/LConn1 -- link3/RConn1
  joint3/RConn4 -- PS-Simulink Converter4/LConn1
  joint3/RConn1 -- link3/LConn1
  joint6/RConn2 -- PS-Simulink Converter11/LConn1
  joint5/RConn4 -- PS-Simulink Converter8/LConn1
  joint3/LConn1 -- link2/RConn1
  joint6/RConn4 -- PS-Simulink Converter10/LConn1
  joint4/LConn2 -- Conn4/RConn1
  joint7/RConn4 -- PS-Simulink Converter12/LConn1
  joint2/LConn2 -- Conn2/RConn1
  joint1/LConn2 -- Conn1/RConn1
  joint1/RConn3 -- PS-Simulink Converter14/LConn1
  PS-Simulink Converter15/LConn1 -- joint2/RConn3
  PS-Simulink Converter16/LConn1 -- joint3/RConn3
  PS-Simulink Converter17/LConn1 -- joint4/RConn3
  PS-Simulink Converter18/LConn1 -- joint5/RConn3
  PS-Simulink Converter19/LConn1 -- joint6/RConn3
  PS-Simulink Converter20/LConn1 -- joint7/RConn3

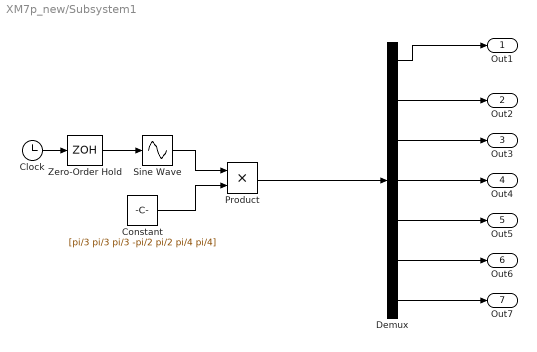
== system XM7p_new/Subsystem1 ==
  Clock : Clock
  Constant : Constant  Value=[pi/3 pi/3 pi/3 -pi/2 pi/2 pi/4 pi/4]
  Demux : Demux  Outputs=7
  Product : Product
  Sine Wave : Sin  TimeSource=Use external signal  Frequency=0.1  SampleTime=0
  Zero-Order Hold : ZeroOrderHold  SampleTime=0.001
  Out1 : Outport
  Out2 : Outport  Port=2
  Out3 : Outport  Port=3
  Out4 : Outport  Port=4
  Out5 : Outport  Port=5
  Out6 : Outport  Port=6
  Out7 : Outport  Port=7
  wires:
  Constant/1 -> Product/2
  Demux/2 -> Out2/1
  Zero-Order Hold/1 -> Sine Wave/1
  Clock/1 -> Zero-Order Hold/1
  Sine Wave/1 -> Product/1
  Demux/5 -> Out5/1
  Product/1 -> Demux/1
  Demux/1 -> Out1/1
  Demux/4 -> Out4/1
  Demux/6 -> Out6/1
  Demux/3 -> Out3/1
  Demux/7 -> Out7/1

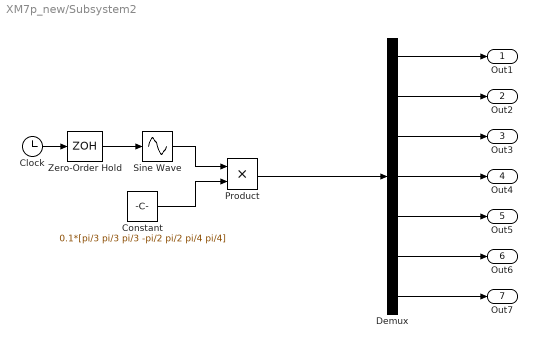
== system XM7p_new/Subsystem2 ==
  Clock : Clock
  Constant : Constant  Value=0.1*[pi/3 pi/3 pi/3 -pi/2 pi/2 pi/4 pi/4]
  Demux : Demux  Outputs=7
  Product : Product
  Sine Wave : Sin  TimeSource=Use external signal  Frequency=0.1  Phase=pi/2  SampleTime=0
  Zero-Order Hold : ZeroOrderHold  SampleTime=0.001
  Out1 : Outport
  Out2 : Outport  Port=2
  Out3 : Outport  Port=3
  Out4 : Outport  Port=4
  Out5 : Outport  Port=5
  Out6 : Outport  Port=6
  Out7 : Outport  Port=7
  wires:
  Constant/1 -> Product/2
  Demux/2 -> Out2/1
  Zero-Order Hold/1 -> Sine Wave/1
  Clock/1 -> Zero-Order Hold/1
  Sine Wave/1 -> Product/1
  Demux/5 -> Out5/1
  Product/1 -> Demux/1
  Demux/1 -> Out1/1
  Demux/4 -> Out4/1
  Demux/6 -> Out6/1
  Demux/3 -> Out3/1
  Demux/7 -> Out7/1

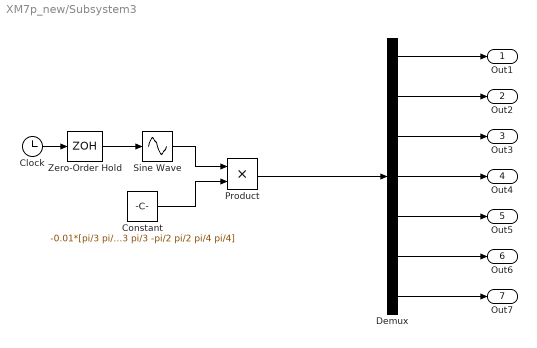
== system XM7p_new/Subsystem3 ==
  Clock : Clock
  Constant : Constant  Value=-0.01*[pi/3 pi/3 pi/3 -pi/2 pi/2 pi/4 pi/4]
  Demux : Demux  Outputs=7
  Product : Product
  Sine Wave : Sin  TimeSource=Use external signal  Frequency=0.1  SampleTime=0
  Zero-Order Hold : ZeroOrderHold  SampleTime=0.001
  Out1 : Outport
  Out2 : Outport  Port=2
  Out3 : Outport  Port=3
  Out4 : Outport  Port=4
  Out5 : Outport  Port=5
  Out6 : Outport  Port=6
  Out7 : Outport  Port=7
  wires:
  Constant/1 -> Product/2
  Demux/2 -> Out2/1
  Zero-Order Hold/1 -> Sine Wave/1
  Clock/1 -> Zero-Order Hold/1
  Sine Wave/1 -> Product/1
  Demux/5 -> Out5/1
  Product/1 -> Demux/1
  Demux/1 -> Out1/1
  Demux/4 -> Out4/1
  Demux/6 -> Out6/1
  Demux/3 -> Out3/1
  Demux/7 -> Out7/1

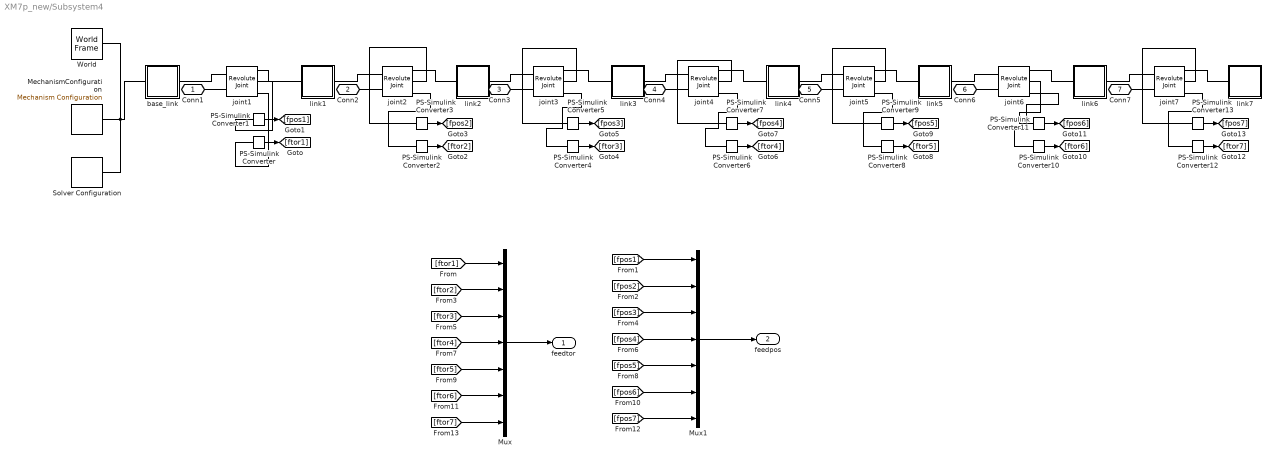
== system XM7p_new/Subsystem4 ==
  MechanismConfiguration : sm_lib/Utilities/Mechanism Configuration  UniformGravity=Constant  GravityVector=[0 0 -9.80665]  GravityVectorUnits=m/s^2  LinearizationDelta=0.001  JointModeTransitionNonlinearIterations=2
  Mux : Mux  Inputs=7
  Mux1 : Mux  Inputs=7
  PS-Simulink Converter{,2,4,6,8,10,12} (7 alike) : nesl_utility/PS-Simulink Converter  PhysicalDomain=network_engine_domain  SubClassName=ps_output  LeftPortType=input  RightPortType=output  PseudoPeriodic=off  Frequencies=[]  VectorFormat=1-D array  Unit=N*m  AffineConversion=off
  PS-Simulink Converter{1,3,5,7,9,11,13} (7 alike) : nesl_utility/PS-Simulink Converter  PhysicalDomain=network_engine_domain  SubClassName=ps_output  LeftPortType=input  RightPortType=output  PseudoPeriodic=off  Frequencies=[]  VectorFormat=1-D array  Unit=rad  AffineConversion=off
  Solver Configuration : nesl_utility/Solver Configuration  PhysicalDomain=network_engine_domain  SubClassName=solver  LeftPortType=input  RightPortType=generic  Tones=[]  Harmonics=[]  SimulateNoise=off  Profile=off  UseLocalSampling=off  EnableSwitchedLinearOptims=on  FrequencyDomain=off  UseCCode=off  RelTol=0.001  AbsTol=1e-06  MinStep=1e-09  ToWorkspace=off  RevertToSquareIcSolve=off  NumHomotopyIterations=100  PhasorMode=off  PhasorModeNumHarmonics=1  ConsistencySolver=NEWTON_FTOL  IndexReductionMethod=DerivativeReplacement  DoDC=off  ResidualTolerance=1e-09  ConsistencyTolSource=GLOBAL  ConsistencyAbsTol=0.001  ConsistencyRelTol=0.001  ConsistencyTolFactor=0.001  UseLocalSolver=off  LocalSolverChoice=NE_BACKWARD_EULER_ADVANCER  ResolveIndetEquations=on  FunctionEvalNumThread=1  LocalSolverSampleTime=0.001  DoFixedCost=off  MaxNonlinIter=3  MaxModeIter=2  ComputeImpulses=off  ImpulseIterations=2  LinearAlgebra=auto  LinearAlgebraNumThread=0  EquationFormulation=NE_TIME_EF  DelaysMemoryBudget=1024  AutomaticFiltering=on  FilteringTimeConstant=0.001  PartitionStorageMethod=AS_NEEDED  PartitionMemoryBudget=1024  PartitionMethod=ROBUST  MultibodyUseLocalSolver=off  MultibodyLocalSolverChoice=ODE1  MultibodyLocalSolverSampleTime=0.001
  World : sm_lib/Frames and Transforms/World Frame
  base_link : Subsystem
  joint1 : sm_lib/Joints/Revolute Joint  JointMode=Normal  CompositeWrenchDir=FollowerOnBase  CompositeWrenchFrame=BaseFrame  SenseConstraintForce=off  SenseConstraintTorque=off  SenseTotalForce=off  SenseTotalTorque=off  PositionTargetSpecify=off  PositionTargetPriority=High  PositionTargetValue=0  PositionTargetValueUnits=deg  VelocityTargetSpecify=off  VelocityTargetPriority=High  VelocityTargetValue=0  VelocityTargetValueUnits=deg/s  EquilibriumPosition=0  EquilibriumPositionUnits=deg  SpringStiffness=0  SpringStiffnessUnits=N*m/deg  DampingCoefficient=0  DampingCoefficientUnits=kg*m^2/(rad*s)  LowerLimitSpecify=on  LowerLimitBound=-2.97  LowerLimitBoundUnits=rad  LowerLimitStiffness=1e4  LowerLimitStiffnessUnits=N*m/deg  LowerLimitDamping=10  LowerLimitDampingUnits=N*m/(deg/s)  LowerLimitTransitionRegionWidth=0.1  LowerLimitTransitionRegionWidthUnits=deg  UpperLimitSpecify=on  UpperLimitBound=2.97  UpperLimitBoundUnits=rad  UpperLimitStiffness=1e4  UpperLimitStiffnessUnits=N*m/deg  UpperLimitDamping=10  UpperLimitDampingUnits=N*m/(deg/s)  UpperLimitTransitionRegionWidth=0.1  UpperLimitTransitionRegionWidthUnits=deg  TorqueActuationMode=ComputedTorque  MotionActuationMode=InputMotion  SensePosition=on  SenseVelocity=off  SenseAcceleration=off  SenseTorqueForce=on  SenseLowerLimitTorqueForce=off  SenseUpperLimitTorqueForce=off
  joint2 : sm_lib/Joints/Revolute Joint  JointMode=Normal  CompositeWrenchDir=FollowerOnBase  CompositeWrenchFrame=BaseFrame  SenseConstraintForce=off  SenseConstraintTorque=off  SenseTotalForce=off  SenseTotalTorque=off  PositionTargetSpecify=off  PositionTargetPriority=High  PositionTargetValue=0  PositionTargetValueUnits=deg  VelocityTargetSpecify=off  VelocityTargetPriority=High  VelocityTargetValue=0  VelocityTargetValueUnits=deg/s  EquilibriumPosition=0  EquilibriumPositionUnits=deg  SpringStiffness=0  SpringStiffnessUnits=N*m/deg  DampingCoefficient=0  DampingCoefficientUnits=kg*m^2/(rad*s)  LowerLimitSpecify=on  LowerLimitBound=-2.09  LowerLimitBoundUnits=rad  LowerLimitStiffness=1e4  LowerLimitStiffnessUnits=N*m/deg  LowerLimitDamping=10  LowerLimitDampingUnits=N*m/(deg/s)  LowerLimitTransitionRegionWidth=0.1  LowerLimitTransitionRegionWidthUnits=deg  UpperLimitSpecify=on  UpperLimitBound=2.09  UpperLimitBoundUnits=rad  UpperLimitStiffness=1e4  UpperLimitStiffnessUnits=N*m/deg  UpperLimitDamping=10  UpperLimitDampingUnits=N*m/(deg/s)  UpperLimitTransitionRegionWidth=0.1  UpperLimitTransitionRegionWidthUnits=deg  TorqueActuationMode=ComputedTorque  MotionActuationMode=InputMotion  SensePosition=on  SenseVelocity=off  SenseAcceleration=off  SenseTorqueForce=on  SenseLowerLimitTorqueForce=off  SenseUpperLimitTorqueForce=off
  joint3 : sm_lib/Joints/Revolute Joint  JointMode=Normal  CompositeWrenchDir=FollowerOnBase  CompositeWrenchFrame=BaseFrame  SenseConstraintForce=off  SenseConstraintTorque=off  SenseTotalForce=off  SenseTotalTorque=off  PositionTargetSpecify=off  PositionTargetPriority=High  PositionTargetValue=0  PositionTargetValueUnits=deg  VelocityTargetSpecify=off  VelocityTargetPriority=High  VelocityTargetValue=0  VelocityTargetValueUnits=deg/s  EquilibriumPosition=0  EquilibriumPositionUnits=deg  SpringStiffness=0  SpringStiffnessUnits=N*m/deg  DampingCoefficient=0  DampingCoefficientUnits=kg*m^2/(rad*s)  LowerLimitSpecify=on  LowerLimitBound=-2.97  LowerLimitBoundUnits=rad  LowerLimitStiffness=1e4  LowerLimitStiffnessUnits=N*m/deg  LowerLimitDamping=10  LowerLimitDampingUnits=N*m/(deg/s)  LowerLimitTransitionRegionWidth=0.1  LowerLimitTransitionRegionWidthUnits=deg  UpperLimitSpecify=on  UpperLimitBound=2.97  UpperLimitBoundUnits=rad  UpperLimitStiffness=1e4  UpperLimitStiffnessUnits=N*m/deg  UpperLimitDamping=10  UpperLimitDampingUnits=N*m/(deg/s)  UpperLimitTransitionRegionWidth=0.1  UpperLimitTransitionRegionWidthUnits=deg  TorqueActuationMode=ComputedTorque  MotionActuationMode=InputMotion  SensePosition=on  SenseVelocity=off  SenseAcceleration=off  SenseTorqueForce=on  SenseLowerLimitTorqueForce=off  SenseUpperLimitTorqueForce=off
  joint4 : sm_lib/Joints/Revolute Joint  JointMode=Normal  CompositeWrenchDir=FollowerOnBase  CompositeWrenchFrame=BaseFrame  SenseConstraintForce=off  SenseConstraintTorque=off  SenseTotalForce=off  SenseTotalTorque=off  PositionTargetSpecify=off  PositionTargetPriority=High  PositionTargetValue=0  PositionTargetValueUnits=deg  VelocityTargetSpecify=off  VelocityTargetPriority=High  VelocityTargetValue=0  VelocityTargetValueUnits=deg/s  EquilibriumPosition=0  EquilibriumPositionUnits=deg  SpringStiffness=0  SpringStiffnessUnits=N*m/deg  DampingCoefficient=0  DampingCoefficientUnits=kg*m^2/(rad*s)  LowerLimitSpecify=on  LowerLimitBound=-2.09  LowerLimitBoundUnits=rad  LowerLimitStiffness=1e4  LowerLimitStiffnessUnits=N*m/deg  LowerLimitDamping=10  LowerLimitDampingUnits=N*m/(deg/s)  LowerLimitTransitionRegionWidth=0.1  LowerLimitTransitionRegionWidthUnits=deg  UpperLimitSpecify=on  UpperLimitBound=2.09  UpperLimitBoundUnits=rad  UpperLimitStiffness=1e4  UpperLimitStiffnessUnits=N*m/deg  UpperLimitDamping=10  UpperLimitDampingUnits=N*m/(deg/s)  UpperLimitTransitionRegionWidth=0.1  UpperLimitTransitionRegionWidthUnits=deg  TorqueActuationMode=ComputedTorque  MotionActuationMode=InputMotion  SensePosition=on  SenseVelocity=off  SenseAcceleration=off  SenseTorqueForce=on  SenseLowerLimitTorqueForce=off  SenseUpperLimitTorqueForce=off
  joint5 : sm_lib/Joints/Revolute Joint  JointMode=Normal  CompositeWrenchDir=FollowerOnBase  CompositeWrenchFrame=BaseFrame  SenseConstraintForce=off  SenseConstraintTorque=off  SenseTotalForce=off  SenseTotalTorque=off  PositionTargetSpecify=off  PositionTargetPriority=High  PositionTargetValue=0  PositionTargetValueUnits=deg  VelocityTargetSpecify=off  VelocityTargetPriority=High  VelocityTargetValue=0  VelocityTargetValueUnits=deg/s  EquilibriumPosition=0  EquilibriumPositionUnits=deg  SpringStiffness=0  SpringStiffnessUnits=N*m/deg  DampingCoefficient=0  DampingCoefficientUnits=kg*m^2/(rad*s)  LowerLimitSpecify=on  LowerLimitBound=-2.97  LowerLimitBoundUnits=rad  LowerLimitStiffness=1e4  LowerLimitStiffnessUnits=N*m/deg  LowerLimitDamping=10  LowerLimitDampingUnits=N*m/(deg/s)  LowerLimitTransitionRegionWidth=0.1  LowerLimitTransitionRegionWidthUnits=deg  UpperLimitSpecify=on  UpperLimitBound=2.97  UpperLimitBoundUnits=rad  UpperLimitStiffness=1e4  UpperLimitStiffnessUnits=N*m/deg  UpperLimitDamping=10  UpperLimitDampingUnits=N*m/(deg/s)  UpperLimitTransitionRegionWidth=0.1  UpperLimitTransitionRegionWidthUnits=deg  TorqueActuationMode=ComputedTorque  MotionActuationMode=InputMotion  SensePosition=on  SenseVelocity=off  SenseAcceleration=off  SenseTorqueForce=on  SenseLowerLimitTorqueForce=off  SenseUpperLimitTorqueForce=off
  joint6 : sm_lib/Joints/Revolute Joint  JointMode=Normal  CompositeWrenchDir=FollowerOnBase  CompositeWrenchFrame=BaseFrame  SenseConstraintForce=off  SenseConstraintTorque=off  SenseTotalForce=off  SenseTotalTorque=off  PositionTargetSpecify=off  PositionTargetPriority=High  PositionTargetValue=0  PositionTargetValueUnits=deg  VelocityTargetSpecify=off  VelocityTargetPriority=High  VelocityTargetValue=0  VelocityTargetValueUnits=deg/s  EquilibriumPosition=0  EquilibriumPositionUnits=deg  SpringStiffness=0  SpringStiffnessUnits=N*m/deg  DampingCoefficient=0  DampingCoefficientUnits=kg*m^2/(rad*s)  LowerLimitSpecify=on  LowerLimitBound=-2.09  LowerLimitBoundUnits=rad  LowerLimitStiffness=1e4  LowerLimitStiffnessUnits=N*m/deg  LowerLimitDamping=10  LowerLimitDampingUnits=N*m/(deg/s)  LowerLimitTransitionRegionWidth=0.1  LowerLimitTransitionRegionWidthUnits=deg  UpperLimitSpecify=on  UpperLimitBound=2.09  UpperLimitBoundUnits=rad  UpperLimitStiffness=1e4  UpperLimitStiffnessUnits=N*m/deg  UpperLimitDamping=10  UpperLimitDampingUnits=N*m/(deg/s)  UpperLimitTransitionRegionWidth=0.1  UpperLimitTransitionRegionWidthUnits=deg  TorqueActuationMode=ComputedTorque  MotionActuationMode=InputMotion  SensePosition=on  SenseVelocity=off  SenseAcceleration=off  SenseTorqueForce=on  SenseLowerLimitTorqueForce=off  SenseUpperLimitTorqueForce=off
  joint7 : sm_lib/Joints/Revolute Joint  JointMode=Normal  CompositeWrenchDir=FollowerOnBase  CompositeWrenchFrame=BaseFrame  SenseConstraintForce=off  SenseConstraintTorque=off  SenseTotalForce=off  SenseTotalTorque=off  PositionTargetSpecify=off  PositionTargetPriority=High  PositionTargetValue=0  PositionTargetValueUnits=deg  VelocityTargetSpecify=off  VelocityTargetPriority=High  VelocityTargetValue=0  VelocityTargetValueUnits=deg/s  EquilibriumPosition=0  EquilibriumPositionUnits=deg  SpringStiffness=0  SpringStiffnessUnits=N*m/deg  DampingCoefficient=0  DampingCoefficientUnits=kg*m^2/(rad*s)  LowerLimitSpecify=on  LowerLimitBound=-6.28  LowerLimitBoundUnits=rad  LowerLimitStiffness=1e4  LowerLimitStiffnessUnits=N*m/deg  LowerLimitDamping=10  LowerLimitDampingUnits=N*m/(deg/s)  LowerLimitTransitionRegionWidth=0.1  LowerLimitTransitionRegionWidthUnits=deg  UpperLimitSpecify=on  UpperLimitBound=6.28  UpperLimitBoundUnits=rad  UpperLimitStiffness=1e4  UpperLimitStiffnessUnits=N*m/deg  UpperLimitDamping=10  UpperLimitDampingUnits=N*m/(deg/s)  UpperLimitTransitionRegionWidth=0.1  UpperLimitTransitionRegionWidthUnits=deg  TorqueActuationMode=ComputedTorque  MotionActuationMode=InputMotion  SensePosition=on  SenseVelocity=off  SenseAcceleration=off  SenseTorqueForce=on  SenseLowerLimitTorqueForce=off  SenseUpperLimitTorqueForce=off
  link1 : Subsystem
  link2 : Subsystem
  link3 : Subsystem
  link4 : Subsystem
  link5 : Subsystem
  link6 : Subsystem
  link7 : Subsystem
  Conn1 : PMIOPort  Side=Left
  Conn2 : PMIOPort  Port=2  Side=Left
  Conn3 : PMIOPort  Port=3  Side=Left
  Conn4 : PMIOPort  Port=4  Side=Left
  Conn5 : PMIOPort  Port=5  Side=Left
  Conn6 : PMIOPort  Port=6  Side=Left
  Conn7 : PMIOPort  Port=7  Side=Left
  feedtor : Outport  Unit=N*m
  feedpos : Outport  Port=2  Unit=rad
  wires:
  [fpos5] -> Mux1/5
  PS-Simulink Converter1/1 -> [fpos1]
  [fpos1] -> Mux1/1
  PS-Simulink Converter11/1 -> [fpos6]
  PS-Simulink Converter10/1 -> [ftor6]
  Mux1/1 -> feedpos/1
  [ftor3] -> Mux/3
  PS-Simulink Converter5/1 -> [fpos3]
  PS-Simulink Converter13/1 -> [fpos7]
  PS-Simulink Converter4/1 -> [ftor3]
  Mux/1 -> feedtor/1
  PS-Simulink Converter2/1 -> [ftor2]
  PS-Simulink Converter/1 -> [ftor1]
  PS-Simulink Converter3/1 -> [fpos2]
  PS-Simulink Converter9/1 -> [fpos5]
  PS-Simulink Converter6/1 -> [ftor4]
  PS-Simulink Converter7/1 -> [fpos4]
  PS-Simulink Converter12/1 -> [ftor7]
  [fpos2] -> Mux1/2
  PS-Simulink Converter8/1 -> [ftor5]
  [ftor4] -> Mux/4
  [fpos6] -> Mux1/6
  [ftor2] -> Mux/2
  [fpos7] -> Mux1/7
  [ftor1] -> Mux/1
  [ftor6] -> Mux/6
  [fpos4] -> Mux1/4
  [fpos3] -> Mux1/3
  [ftor7] -> Mux/7
  [ftor5] -> Mux/5
  connections:
  joint4/RConn1 -- link4/LConn1
  joint3/RConn2 -- PS-Simulink Converter5/LConn1
  joint5/RConn1 -- link5/LConn1
  joint1/RConn2 -- PS-Simulink Converter1/LConn1
  joint5/LConn1 -- link4/RConn1
  joint5/RConn2 -- PS-Simulink Converter9/LConn1
  joint2/RConn2 -- PS-Simulink Converter3/LConn1
  joint6/LConn2 -- Conn6/RConn1
  joint1/RConn1 -- link1/LConn1
  joint1/RConn3 -- PS-Simulink Converter/LConn1
  joint2/RConn3 -- PS-Simulink Converter2/LConn1
  joint7/RConn1 -- link7/LConn1
  joint4/RConn3 -- PS-Simulink Converter6/LConn1
  joint5/LConn2 -- Conn5/RConn1
  World/RConn1 -- MechanismConfiguration/RConn1 -- Solver Configuration/RConn1 -- base_link/LConn1
  joint2/LConn1 -- link1/RConn1
  joint7/RConn2 -- PS-Simulink Converter13/LConn1
  joint4/RConn2 -- PS-Simulink Converter7/LConn1
  joint2/RConn1 -- link2/LConn1
  joint7/LConn2 -- Conn7/RConn1
  joint6/RConn1 -- link6/LConn1
  joint6/LConn1 -- link5/RConn1
  joint7/LConn1 -- link6/RConn1
  base_link/RConn1 -- joint1/LConn1
  joint3/LConn2 -- Conn3/RConn1
  joint4/LConn1 -- link3/RConn1
  joint3/RConn3 -- PS-Simulink Converter4/LConn1
  joint3/RConn1 -- link3/LConn1
  joint6/RConn2 -- PS-Simulink Converter11/LConn1
  joint5/RConn3 -- PS-Simulink Converter8/LConn1
  joint3/LConn1 -- link2/RConn1
  joint6/RConn3 -- PS-Simulink Converter10/LConn1
  joint4/LConn2 -- Conn4/RConn1
  joint7/RConn3 -- PS-Simulink Converter12/LConn1
  joint2/LConn2 -- Conn2/RConn1
  joint1/LConn2 -- Conn1/RConn1
